simulink model "PMSM_FOC_Traction"  (R2020b)
settings: Solver=FixedStepAuto  StartTime=0.0  StopTime=10  RelTol=1e-3
model workspace (MAT data in the model file):
  wc : Simulink.Parameter (value not decoded)
values from neighbouring files (symbols this model uses):
  CL_Param = tmp_CL_Param    [PMSM_Parameters.m]
  Cosine_table = [1,0.999995293095708,0.999990587122738,0.999985881149769,0.999981174245477,0.999967055395246,0.999952936545014,0.999938818626106,0.999924698844552,0.999901168979704,0.999877639114857,0.999854108318687,0.999830577522516,0.999797635711730,0.999764694832265,0.999731753021479,0.999698810279369,0.999656459316611,0.999614108353853,0.999571758322418,0.999529405497015,0.999477646313608,0.999425887130201,0 ...(+75635 chars)    [Motor_Table.m]
  ctrlParamsPI = tmp_ctrlParamsPI    [PMSM_Parameters.m]
  Flux_weak = tmp_Fluxweak_struct    [PMSM_Parameters.m]
  FluxObsever = tmp_FluxObsever_struct    [PMSM_Parameters.m]
  Hall_Parameter = tmp_Hall_struct    [PMSM_Parameters.m]
  HFI = tmp_HFI_struct    [PMSM_Parameters.m]
  inverter = struct    [PMSM_Parameters.m]
  MTPA_id_table = [-1.39452500000000,-1.36697494250000,-1.33970177000000,-1.31270548250000,-1.28598608000000,-1.25954356250000,-1.23337793000000,-1.20748918250000,-1.18187732000000,-1.15654234250000,-1.13148425000000,-1.10670304250000,-1.08219872000000,-1.05797128250000,-1.03402073000000,-1.01034706250000,-0.986950280000000,-0.963830382500000,-0.940987370000000,-0.918421242500000,-0.896132000000000,-0.8741196425000 ...(+3439 chars)    [Motor_Table.m]
  MTPA_iq_table = [-10.2740250000000,-10.1791705677750,-10.0840783722000,-9.98875081492500,-9.89319029760000,-9.79739922187500,-9.70137998940000,-9.60513500182500,-9.50866666080000,-9.41197736797500,-9.31506952500000,-9.21794553352500,-9.12060779520000,-9.02305871167500,-8.92530068460000,-8.82733611562500,-8.72916740640000,-8.63079695857500,-8.53222717380000,-8.43346045372500,-8.33449920000000,-8.23534581427500,-8. ...(+3121 chars)    [Motor_Table.m]
  MTPA_Te_Max = single(1.50)    [Motor_Table.m]
  MTPA_Te_Min = single(-1.50)    [Motor_Table.m]
  OPL_Param = tmp_OPL_Param    [PMSM_Parameters.m]
  pmsm = struct    [PMSM_Parameters.m]
  Resolver_Parameter = tmp_Resolver_struct    [PMSM_Parameters.m]
  Sine_table = [0,0.00153398793190718,0.00306797679513693,0.00460196565836668,0.00613595545291901,0.00766988657414913,0.00920381769537926,0.0107377488166094,0.0122716808691621,0.0138054965063930,0.0153393121436238,0.0168731296434999,0.0184069443494082,0.0199405867606401,0.0214742291718721,0.0230078706517816,0.0245415139943361,0.0260749254375696,0.0276083368808031,0.0291417483240366,0.0306751597672701,0.032208281 ...(+75648 chars)    [Motor_Table.m]
  SMO = temp_SMO    [PMSM_Parameters.m]
undefined symbols (not defined in the file or in its folder): DiscIntNeverNeededParam, Kiv, Kiw, Kpv, Kpw, magnitude, sigbuilder_block, SVPWM, Vdc
libraries: powerlib x29, fl_lib x18, simulink x7, nesl_utility x7, pid_lib x5, dspstat3 x4, eeGeneralControl x4, eeDiscretePi x2, powerlib_extras x1, ee_lib x1
(part 3 of 6)

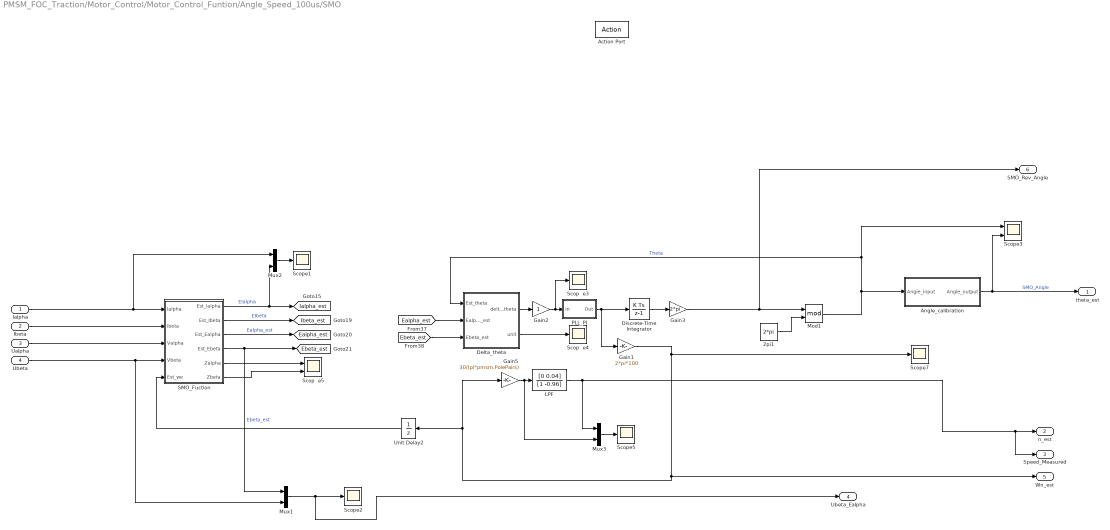
== system PMSM_FOC_Traction/Motor_Control/Motor_Control_Funtion/Angle_Speed_100us/SMO ==
  Ialpha : Inport
  Ibeta : Inport  Port=2
  Ualpha : Inport  Port=3
  Ubeta : Inport  Port=4
  Action Port : ActionPort  ActionPortLabel=if(u1==1)
  2pi1 : Constant  Value=2*pi  OutDataTypeStr=single
  Angle_calibration : Subsystem  TreatAsAtomicUnit=on
      settings: RTWSystemCode=Nonreusable function  RTWFcnNameOpts=Use subsystem name
  Delta_theta : Subsystem  TreatAsAtomicUnit=on
      settings: RTWSystemCode=Nonreusable function  RTWFcnNameOpts=Use subsystem name
  Discrete-Time Integrator : DiscreteIntegrator  gainval=100  SampleTime=-1  ICPrevOutput=DiscIntNeverNeededParam  ICPrevScaledInput=DiscIntNeverNeededParam
  Gain1 : Gain  Gain=2*pi*100  OutDataTypeStr=single
  Gain2 : Gain
  Gain3 : Gain  Gain=2*pi  OutDataTypeStr=single
  Gain5 : Gain  Gain=30/(pi*pmsm.PolePairs)
  LPF : DiscreteFilter  Numerator=[0 0.04]  Denominator=[1 -0.96]
  Mod1 : Math  Operator=mod  SaturateOnIntegerOverflow=on
  Mux1 : Mux  Inputs=2
  Mux2 : Mux  Inputs=2
  Mux3 : Mux  Inputs=2
  PLL_PI : Subsystem  mask{kp=SMO.PLL_KP, ki=SMO.PLL_Ki, Ts=-1}
  SMO_Fuction : Subsystem  mask{A=SMO.A, B=SMO.B, C=SMO.C, k=SMO.k, m=SMO.m, tao=SMO.tao, Ts=inverter.Ts}
  Scop  e3 : Scope
  Scop  e4 : Scope
  Scop  e5 : Scope  NumInputPorts=2
  Scope{1..2,5,7} (4 alike) : Scope
  Scope3 : Scope  NumInputPorts=2
  Unit Delay2 : UnitDelay  SampleTime=-1  HasFrameUpgradeWarning=on
  theta_est : Outport
  n_est : Outport  Port=2
  Speed_Measured : Outport  Port=3
  Ubeta_Ealpha : Outport  Port=4
  Wn_est : Outport  Port=5
  SMO_Rev_Angle : Outport  Port=6
  tag scope: Ealpha_est=global, Ebeta_est=global, Ialpha_est=global, Ibeta_est=global
  wires:
  SMO_Fuction/3(Est_Ealpha) -> [Ealpha_est]  "Ealpha_est"
  SMO_Fuction/6(Zbeta) -> Scop  e5/2
  SMO_Fuction/1(Est_Ialpha) -> Mux2/2, [Ialpha_est]  "EIalpha"
  SMO_Fuction/4(Est_Ebeta) -> Mux1/1, [Ebeta_est]  "Ebeta_est"
  SMO_Fuction/5(Zalpha) -> Scop  e5/1
  SMO_Fuction/2(Est_Ibeta) -> [Ibeta_est]  "EIbeta"
  Mux2/1 -> Scope1/1
  [Ebeta_est] -> Delta_theta/3(Ebeta_est)
  Delta_theta/1(delta_theta) -> Gain2/1
  Gain2/1 -> Scop  e3/1, PLL_PI/1(in)
  [Ealpha_est] -> Delta_theta/2(Ealpha_est)
  Discrete-Time Integrator/1 -> Gain3/1
  Mod1/1 -> Delta_theta/1(Est_theta), Scope3/1, Angle_calibration/1(Angle_input)  "Theta"
  PLL_PI/1(Out) -> Discrete-Time Integrator/1, Gain1/1
  2pi1/1 -> Mod1/2
  Mux3/1 -> Scope5/1
  Delta_theta/2(unit) -> Scop  e4/1
  Gain5/1 -> Mux3/2, LPF/1
  LPF/1 -> Speed_Measured/1, n_est/1, Mux3/1
  Angle_calibration/1(Angle_output) -> theta_est/1, Scope3/2  "SMO_Angle"
  Ialpha/1 -> SMO_Fuction/1(Ialpha), Mux2/1
  Ibeta/1 -> SMO_Fuction/2(Ibeta)
  Ualpha/1 -> SMO_Fuction/3(Valpha)
  Ubeta/1 -> SMO_Fuction/4(Vbeta), Mux1/2
  Gain1/1 -> Wn_est/1, Gain5/1, Unit Delay2/1, Scope7/1
  Mux1/1 -> Ubeta_Ealpha/1, Scope2/1
  Unit Delay2/1 -> SMO_Fuction/5(Est_we)
  Gain3/1 -> SMO_Rev_Angle/1, Mod1/1

== system PMSM_FOC_Traction/Motor_Control/Motor_Control_Funtion/Angle_Speed_100us/SpeedAndAngle ==
  Counter : Inport
  Hall : Inport  Port=2
  Action Port : ActionPort  ActionPortLabel=if(u1==1)
  ACC_OMG : Subsystem  TreatAsAtomicUnit=on
      settings: RTWSystemCode=Nonreusable function  RTWFcnNameOpts=Use subsystem name
  ADC_IRQ : Subsystem  TreatAsAtomicUnit=on
      settings: RTWSystemCode=Nonreusable function  RTWFcnNameOpts=Use subsystem name
  Chart : Stateflow chart  TreatAsAtomicUnit=on
  Scope : Scope
  Subsystem : Subsystem
  Subsystem1 : Subsystem
  Hall_Angle : Outport
  Hall_Speed_RPM : Outport  Port=2
  We : Outport  Port=3
  Gate : Outport  Port=4  VectorParamsAs1DForOutWhenUnconnected=off
  Duty : Outport  Port=5  VectorParamsAs1DForOutWhenUnconnected=off
  BLDC_State : Outport  Port=6  VectorParamsAs1DForOutWhenUnconnected=off
  wires:
  ACC_OMG/4(Counter) -> ADC_IRQ/4(Counter_Hall_IRQ)
  ACC_OMG/2(Acc) -> ADC_IRQ/2(Acc)
  ACC_OMG/3(OMG) -> [Hall_We], We/1, ADC_IRQ/3(OMG)
  ACC_OMG/1(Hall_SpeedRPM) -> Hall_Speed_RPM/1
  ACC_OMG/5(Six_theta) -> ADC_IRQ/5(Six_theta)
  Counter/1 -> ADC_IRQ/1(Counter_ADC_IRQ), ACC_OMG/1(Timer_Counter)
  ADC_IRQ/1(Hall_Angle) -> Hall_Angle/1, Scope/1
  Hall/1 -> Subsystem/2(Hall), ACC_OMG/2(Hall), ACC_OMG/Trigger
  Chart/1(BLDC_State) -> ACC_OMG/3(BLDC_State), Subsystem/1(BLDC_State), BLDC_State/1, Subsystem1/5(BLDC_State)
  Subsystem/2(Duty_Set) -> Subsystem1/2(Lock_Duty)
  ACC_OMG/6(Gate) -> Subsystem1/3(Hall_Gate)
  ACC_OMG/7(Tabc) -> Subsystem1/4(Hall_Duty)
  Subsystem/1(Gate) -> Subsystem1/1(Lock_Gate)
  Subsystem1/1(Gate) -> Gate/1
  Subsystem1/2(Tabc) -> Duty/1

== system PMSM_FOC_Traction/Motor_Control/Motor_Control_Funtion/Angle_Speed_100us/Speed_Angle_Selector ==
  Resolver_Speed : Inport
  Resolver_Angle : Inport  Port=2
  Resolver_PLL_Speed : Inport  Port=3
  Resolver_PLL_Angle : Inport  Port=4
  Sensorless_Speed : Inport  Port=5
  Sensorless_Angle : Inport  Port=6
  Hall_Speed : Inport  Port=7
  Hall_Angle : Inport  Port=8
  Hall : Subsystem
  Hall_Angle_Enable : Constant  Value=Hall_Parameter.Angle_Enable  OutDataTypeStr=uint8
  If1 : If  IfExpression=u1==1  ShowElse=off
  If2 : If  NumInputs=2  IfExpression=u1==1 | u2==1  ShowElse=off
  If3 : If  IfExpression=u1==1  ShowElse=off
  If5 : If  IfExpression=u1==1  ShowElse=off
  Merge : Merge  Inputs=4
  Merge1 : Merge  Inputs=4
  Resolver_Dir : Subsystem
  Resolver_Enable : Constant  Value=Resolver_Parameter.Angle_Enable  OutDataTypeStr=uint8
  Resolver_PLL : Subsystem
  Resolver_PLL_Enable : Constant  Value=Resolver_Parameter.PLL_Angle_Enable  OutDataTypeStr=uint8
  Sensorless : Subsystem
  Sensorless_Enable : Constant  Value=OPL_Param.Func_Enable  OutDataTypeStr=uint8
  Sensorless_Enable1 : Constant  Value=FluxObsever.Angle_Enable  OutDataTypeStr=uint8
  Speed : Outport
  Theta : Outport  Port=2
  wires:
  If5/1 -> Resolver_Dir/Action
  Resolver_Enable/1 -> If5/1
  Hall_Speed/1 -> Hall/1(In1)
  Hall_Angle/1 -> Hall/2(In2)
  Sensorless_Speed/1 -> Sensorless/1(In1)
  Sensorless_Angle/1 -> Sensorless/2(In2)
  Resolver_Speed/1 -> Resolver_Dir/1(In1)
  Resolver_Angle/1 -> Resolver_Dir/2(In2)
  Resolver_PLL_Speed/1 -> Resolver_PLL/1(In1)
  Resolver_PLL_Angle/1 -> Resolver_PLL/2(In2)
  If1/1 -> Resolver_PLL/Action
  Resolver_PLL_Enable/1 -> If1/1
  Sensorless_Enable/1 -> If2/1
  If2/1 -> Sensorless/Action
  Hall_Angle_Enable/1 -> If3/1
  If3/1 -> Hall/Action
  Resolver_Dir/1(Out1) -> Merge/1
  Resolver_PLL/1(Out1) -> Merge/2
  Sensorless/1(Out1) -> Merge/3
  Hall/1(Out1) -> Merge/4
  Resolver_Dir/2(Out2) -> Merge1/1
  Resolver_PLL/2(Out2) -> Merge1/2
  Sensorless/2(Out2) -> Merge1/3
  Hall/2(Out2) -> Merge1/4
  Merge1/1 -> Theta/1
  Merge/1 -> Speed/1
  Sensorless_Enable1/1 -> If2/2

== system PMSM_FOC_Traction/Motor_Control/Motor_Control_Funtion/Angle_Speed_100us/Speed_Resolver ==
  Theta : Inport
  Action Port : ActionPort  ActionPortLabel=if(u1==1)
  DT2 : DataTypeConversion  OutDataTypeStr=single
  Scope : Scope
  Scope1 : Scope
  Speed_cacl : Subsystem  TreatAsAtomicUnit=on
      settings: RTWSystemCode=Nonreusable function  RTWFcnNameOpts=Use subsystem name
  Speed_out : Outport
  Dir_Angle : Outport  Port=2
  wires:
  Theta/1 -> DT2/1, Speed_cacl/1(position)  "Theta_input"
  Speed_cacl/1(Speed_RPM) -> Scope1/1, Speed_out/1  "Speed_RPM_Filtered"
  DT2/1 -> Scope/1, Dir_Angle/1  "Direct_Angle"

== system PMSM_FOC_Traction/Motor_Control/Motor_Control_Funtion/Angle_Speed_100us/Startup_OPL ==
  OPL_Torque : Inport
  OPL_State : Inport  Port=2
  Smo_theta : Inport  Port=3
  Action Port : ActionPort  ActionPortLabel=if(u1==2|u1==3 | u1==3)
  If2 : If  IfExpression=u1==2  ElseIfExpressions=u1==3  ShowElse=off
  Merge : Merge
  Merge1 : Merge
  OPL_SpeedRPM : Constant  Value=OPL_Param.Target_RPM
  Scope3 : Scope  NumInputPorts=3
  Subsystem : Subsystem
  Subsystem1 : Subsystem
  Force_Angle : Outport
  OPL_Torque_Com : Outport  Port=2
  wires:
  OPL_State/1 -> If2/1
  If2/1 -> Subsystem/Action
  OPL_Torque/1 -> Subsystem1/1(OPL_Torque), Subsystem/2(OPL_Torque)
  If2/2 -> Subsystem1/Action
  Subsystem/1(Force_Angle) -> Merge/1
  Subsystem1/1(Force_Angle) -> Merge/2
  Merge/1 -> Force_Angle/1
  Subsystem/2(OPL_Torque_Com) -> Merge1/1
  Subsystem1/2(OPL_Torque_Com) -> Merge1/2
  Merge1/1 -> OPL_Torque_Com/1
  OPL_SpeedRPM/1 -> Subsystem1/3(Force_RPM), Subsystem/1(OPL_Speed)
  Smo_theta/1 -> Scope3/2, Subsystem/3(Smo_theta)
  Subsystem/3(Delta_theta) -> Subsystem1/2(Delta_theta)
  Subsystem/4(Force_Switch) -> Scope3/3, Subsystem1/4(Force_Switch)
  Subsystem1/3(Force_Angle1) -> Scope3/1

== system PMSM_FOC_Traction/Motor_Control/Motor_Control_Funtion/Angle_Speed_100us/Subsystem ==
  Action Port : ActionPort  ActionPortLabel=if((u1==1)&(u2==1))
  Sensorless_Enable : Constant  OutDataTypeStr=boolean
  Out1 : Outport
  wires:
  Sensorless_Enable/1 -> Out1/1

== system PMSM_FOC_Traction/Motor_Control/Motor_Control_Funtion/Angle_Speed_100us/Subsystem1 ==
  Action Port : ActionPort  ActionPortLabel=else
  Sensorless_Disable : Constant  Value=0  OutDataTypeStr=boolean
  Out1 : Outport
  wires:
  Sensorless_Disable/1 -> Out1/1

== system PMSM_FOC_Traction/Motor_Control/Motor_Control_Funtion/Control_Command_2ms/Speed_PI ==
  Speed_Command : Inport
  Speed_Measured : Inport  Port=2
  HFI_State : Inport  Port=3
  Motor_State : Inport  Port=4
  BLDC_State : Inport  Port=5
  Action Port : ActionPort  ActionPortLabel=case [ 1 ]:
  Add2 : Sum  Inputs=|+-
  Hall_Enalble : Constant  Value=Hall_Parameter.BLDC_Start  OutDataTypeStr=uint8
  If1 : If  NumInputs=2  IfExpression=(u1==1)&(u2==3)|(u1~=1)  ShowElse=off
  Scope2 : Scope
  Speed_PI : Subsystem
  Iq_ref : Outport  VectorParamsAs1DForOutWhenUnconnected=off
  wires:
  Speed_Command/1 -> Add2/1
  Speed_Measured/1 -> Add2/2
  Add2/1 -> Speed_PI/1(PI_input)  "currentControlError"
  Speed_PI/1(PI_out) -> Iq_ref/1, Scope2/1
  HFI_State/1 -> Speed_PI/2(HFI_State)
  Motor_State/1 -> Speed_PI/3(Motor_State)
  BLDC_State/1 -> If1/2
  Hall_Enalble/1 -> If1/1
  If1/1 -> Speed_PI/Action

== system PMSM_FOC_Traction/Motor_Control/Motor_Control_Funtion/Control_Command_2ms/Switch Case Action Subsystem ==
  Iq_in : Inport
  Action Port : ActionPort  ActionPortLabel=case [ 2 ]:
  Iq_out : Outport
  wires:
  Iq_in/1 -> Iq_out/1

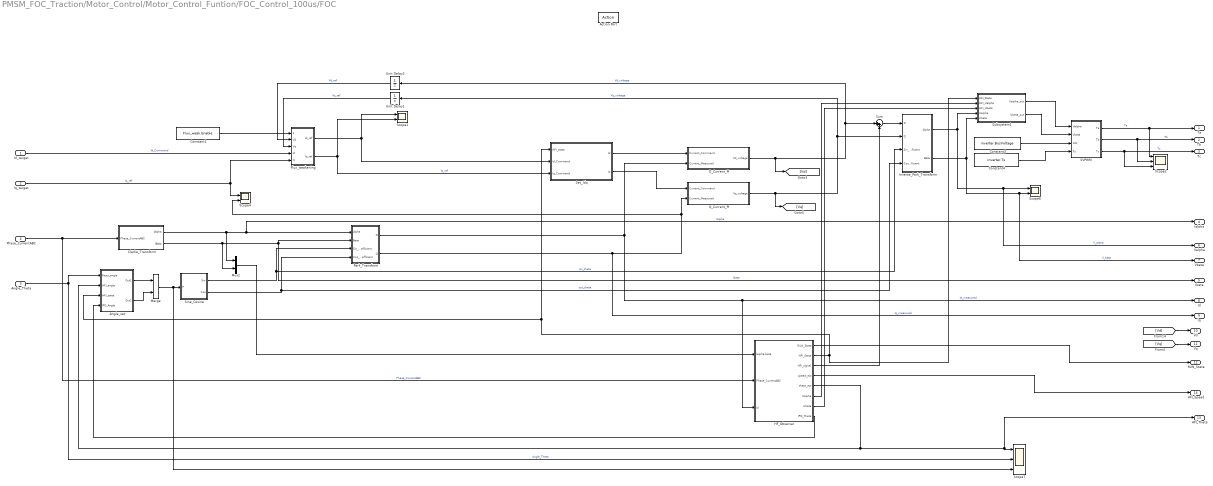
== system PMSM_FOC_Traction/Motor_Control/Motor_Control_Funtion/FOC_Control_100us/FOC ==
  Id_target : Inport
  Iq_target : Inport  Port=2
  Angle_Theta : Inport  Port=3  OutMin=0  OutMax=2*pi
  Phase_CurrentABC : Inport  Port=4  PortDimensions=3
  Action Port : ActionPort  ActionPortLabel=if((u1==1)&(u2==3)|(u1~=1))
  Angle_set : Subsystem  TreatAsAtomicUnit=on
      settings: RTWSystemCode=Nonreusable function  RTWFcnNameOpts=Use subsystem name
  Clarke_Transform : Subsystem  TreatAsAtomicUnit=on
      settings: RTWSystemCode=Nonreusable function  RTWFcnNameOpts=Use subsystem name
  Constant1 : Constant  Value=Flux_weak.Enable  OutDataTypeStr=single
  Constant3 : Constant  Value=inverter.BusVoltage  OutDataTypeStr=single
  Constant4 : Constant  Value=inverter.Ts  OutDataTypeStr=single
  D_Current_PI : Subsystem  TreatAsAtomicUnit=on
      settings: RTWSystemCode=Nonreusable function  RTWFcnNameOpts=Use subsystem name
  "Flux_weakening " : Subsystem
  HF_Observer : Subsystem  TreatAsAtomicUnit=on
      settings: RTWSystemCode=Nonreusable function  RTWFcnNameOpts=Use subsystem name  RTWFileNameOpts=Use subsystem name
  Inverse_Park_Transform : Subsystem  TreatAsAtomicUnit=on
      settings: RTWSystemCode=Nonreusable function  RTWFcnNameOpts=Use subsystem name
      mask Display:
      | port_label('input',1,'D')
      | port_label('input',2,'Q')
      | port_label('input',3,'Sin')
      | port_label('input',4,'Cos')
      | port_label('output',1,'\alpha','texmode', 'on')
      | port_label('output',2,'\beta','texmode', 'on')
  Merge : Merge
  Mux2 : Mux  Inputs=2
  Park_Transform : Subsystem  TreatAsAtomicUnit=on
      settings: RTWSystemCode=Nonreusable function  RTWFcnNameOpts=Use subsystem name
      mask Display:
      | port_label('input',1,'\alpha','texmode', 'on')
      | port_label('input',2,'\beta','texmode', 'on')
      | port_label('input',3,'Sin')
      | port_label('input',4,'Cos')
      | port_label('output',1,'D')
      | port_label('output',2,'Q')
  Q_Current_PI : Subsystem  TreatAsAtomicUnit=on
      settings: RTWSystemCode=Nonreusable function  RTWFcnNameOpts=Use subsystem name
  SVPWM : Subsystem  AncestorBlock=SVPWM/SVPWM  TreatAsAtomicUnit=on  RTWFcnName=SVPWM  RTWFileName=SVPWM
      settings: RTWSystemCode=Nonreusable function  RTWFcnNameOpts=Use subsystem name
      mask Display:
      | plot([0.000 0.020 0.041 0.061 0.082 0.102 0.122 0.143 0.163 0.184 0.204 0.224 0.245 0.265 0.286 0.306 0.327 0.347 0.367 0.388 0.408 0.429 0.449 0.469 0.490 0.510 0.531 0.551 0.571 0.592 0.612 0.633 0.653 0.673 0.694 0.714 0.735 0.755 0.776 0.796 0.816 0.837 0.857 0.878 0.898 0.918 0.939 0.959 0.980 1.000 ], ...
      |      [0.500 0.586 0.671 0.753 0.831 0.858 0.875 0.885 0.890 0.887 0.879 0.864 0.844 0.855 0.872 0.884 0.889 0.888 0.881 0.867 0.847 0.793 0.713 0.629 0.543 0.457 0.371 0.287 0.207 0.153 0.133 0.119 0.112 0.111 0.116 0.128 0.145 0.156 0.136 0.121 0.113 0.110 0.115 0.125 0.142 0.169 0.247 0.329 0.414 0.500 ])
  Scope1 : Scope  NumInputPorts=2
  Scope2 : Scope  NumInputPorts=3
  Scope4 : Scope  NumInputPorts=2
  Scope6 : Scope  NumInputPorts=2
  Scope7 : Scope  NumInputPorts=3
  Set_Idq : Subsystem  TreatAsAtomicUnit=on
      settings: RTWSystemCode=Nonreusable function  RTWFcnNameOpts=Use subsystem name
  Sine_Cosine : Subsystem  TreatAsAtomicUnit=on
      settings: RTWSystemCode=Nonreusable function  RTWFcnNameOpts=Use subsystem name
  Subsystem1 : Subsystem
  Sum : Sum  Inputs=|++
  Unit Delay1 : UnitDelay  SampleTime=-1  HasFrameUpgradeWarning=on
  Unit Delay2 : UnitDelay  SampleTime=-1  HasFrameUpgradeWarning=on
  Ta : Outport
  Tb : Outport  Port=2
  Tc : Outport  Port=3
  Ialpha : Outport  Port=4
  Ibeta : Outport  Port=5
  Valpha : Outport  Port=6
  Vbeta : Outport  Port=7
  Id : Outport  Port=8
  Iq : Outport  Port=9
  Vd : Outport  Port=10
  Vq : Outport  Port=11
  RUN_State : Outport  Port=12
  HFI_Theta : Outport  Port=13
  HFI_Speed : Outport  Port=14
  wires:
  Park_Transform/1(D) -> HF_Observer/3(Id), Id/1, D_Current_PI/2(Current_Measured)  "Id_measured"
  Constant4/1 -> SVPWM/4(Ts)
  SVPWM/3(Tc) -> Tc/1, Scope2/3  "Tc"
  SVPWM/2(Tb) -> Scope2/2, Tb/1  "Tb"
  Park_Transform/2(Q) -> Iq/1, Scope4/2, Q_Current_PI/2(Current_Measured)  "Iq_measured"
  Sine_Cosine/2(Cos) -> Park_Transform/4(Cos_Coefficient), Inverse_Park_Transform/4(Cos_Coefficient)  "cos_theta"
  Sine_Cosine/1(Sin) -> Park_Transform/3(Sin_Coefficient), Inverse_Park_Transform/3(Sin_Coefficient)  "sin_theta"
  Constant3/1 -> SVPWM/3(Vdc)
  D_Current_PI/1(Vd_voltage) -> [Vd], Unit Delay2/1, Sum/1  "Vd_voltage"
  Q_Current_PI/1(Vq_voltage) -> [Vq], Unit Delay1/1, Inverse_Park_Transform/2(Q)  "Vq_voltage"
  SVPWM/1(Ta) -> Scope2/1, Ta/1  "Ta"
  Id_target/1 -> "Flux_weakening "/4(Id)  "Id_Command"
  Iq_target/1 -> "Flux_weakening "/5(Iq), Scope4/1  "Iq_ref"
  Clarke_Transform/2(IBeta) -> Mux2/2, Ibeta/1, Park_Transform/2(Beta)  "Ibeta"
  Clarke_Transform/1(IAlpha) -> Ialpha/1, Park_Transform/1(Alpha), Mux2/1  "Ialpha"
  Unit Delay2/1 -> "Flux_weakening "/2(Vd)  "Vd_ref"
  Unit Delay1/1 -> "Flux_weakening "/3(Vq)  "Vq_ref"
  "Flux_weakening "/1(Id_ref) -> Scope1/1, Set_Idq/2(Id_Command)
  "Flux_weakening "/2(Iq_ref) -> Set_Idq/3(Iq_Command), Scope1/2  "Iq_ref"
  Constant1/1 -> "Flux_weakening "/1(Enable)
  Inverse_Park_Transform/1(Alpha) -> Scope6/1, Valpha/1, Subsystem1/4(Ualpha)  "V_alpha"
  Inverse_Park_Transform/2(Beta) -> Scope6/2, Vbeta/1, Subsystem1/5(Ubeta)  "V_beta"
  Phase_CurrentABC/1 -> HF_Observer/2(Phase_CurrentABC), Clarke_Transform/1(Phase_CurrentABC)  "Phase_CurrentABC"
  Sum/1 -> Inverse_Park_Transform/1(D)
  HF_Observer/3(HFI_signal) -> Sum/2
  HF_Observer/4(speed_est) -> HFI_Speed/1
  Angle_Theta/1 -> Scope7/2, Angle_set/1(Reso_angle)  "Angle_Theta"
  Mux2/1 -> HF_Observer/1(Ialpha-beta)
  HF_Observer/5(theta_est) -> HFI_Theta/1, Scope7/1, Angle_set/2(HFI_angle)
  Merge/1 -> Scope7/3, Sine_Cosine/1(P)
  Angle_set/1(Out1) -> Merge/1
  Angle_set/2(Out2) -> Merge/2
  Subsystem1/1(Ualpha_out) -> SVPWM/1(Valpha)
  Subsystem1/2(Ubeta_out) -> SVPWM/2(Vbeta)
  HF_Observer/6(Ualpha) -> Subsystem1/2(HFI_Ualpha)
  HF_Observer/7(Ubeta) -> Subsystem1/3(HFI_Ubeta)
  HF_Observer/2(HFI_State) -> Subsystem1/1(HFI_State), Set_Idq/1(HFI_state), Angle_set/3(HFI_state)
  HF_Observer/1(RUN_State) -> RUN_State/1
  Set_Idq/1(Id) -> D_Current_PI/1(Current_Command)
  Set_Idq/2(Iq) -> Q_Current_PI/1(Current_Command)
  HF_Observer/8(IPD_Theta) -> Angle_set/4(IPD_Angle)
  [Vq] -> Vq/1
  [Vd] -> Vd/1

== system PMSM_FOC_Traction/Motor_Control/Motor_Control_Funtion/FOC_Control_100us/Iq_selector ==
  Motor_state : Inport
  PI_IQ : Inport  Port=2
  OPL_IQ : Inport  Port=3
  If1 : If  IfExpression=u1 ==2 | u1 ==3
  Merge : Merge
  Subsystem : Subsystem
  Subsystem1 : Subsystem
  Iq_ref : Outport
  wires:
  Motor_state/1 -> If1/1
  If1/1 -> Subsystem/Action
  OPL_IQ/1 -> Subsystem/1(In1)
  PI_IQ/1 -> Subsystem1/1(In1)
  Subsystem/1(Out1) -> Merge/1
  Subsystem1/1(Out1) -> Merge/2
  Merge/1 -> Iq_ref/1
  If1/2 -> Subsystem1/Action

== system PMSM_FOC_Traction/Motor_Control/Motor_Control_Funtion/FOC_Control_100us/MTPA ==
  Te_ref : Inport
  1-D Lookup Table4 : Lookup_n-D  NumberOfTableDimensions=1  LookupTableObject=''  BreakpointsForDimension1=single(linspace(MTPA_Te_Min,MTPA_Te_Max,length(MTPA_id_table)));  BreakpointsForDimension1FirstPoint=10  BreakpointsForDimension2FirstPoint=10  BreakpointsForDimension1Spacing=12  BreakpointsForDimension2Spacing=12  IndexSearchMethod=Evenly spaced points  Table=MTPA_id_table  InterpMethod=Flat  DiagnosticForOutOfRangeInput=Error  InternalRulePriority=Speed  RndMeth=Simplest  InputSameDT=on
  1-D Lookup Table5 : Lookup_n-D  NumberOfTableDimensions=1  LookupTableObject=''  BreakpointsForDimension1=single(linspace(MTPA_Te_Min,MTPA_Te_Max,length(MTPA_id_table)));  BreakpointsForDimension1FirstPoint=10  BreakpointsForDimension2FirstPoint=10  BreakpointsForDimension1Spacing=12  BreakpointsForDimension2Spacing=12  IndexSearchMethod=Evenly spaced points  Table=MTPA_iq_table  InterpMethod=Flat  DiagnosticForOutOfRangeInput=Error  InternalRulePriority=Speed  RndMeth=Simplest  InputSameDT=on
  Saturation : Saturate  UpperLimit=MTPA_Te_Max-0.01  LowerLimit=MTPA_Te_Min+0.01
  Saturation1 : Saturate  UpperLimit=MTPA_Te_Max-0.01  LowerLimit=MTPA_Te_Min+0.01
  Id_ref : Outport
  Iq_ref : Outport  Port=2
  wires:
  Te_ref/1 -> Saturation1/1, Saturation/1
  Saturation/1 -> 1-D Lookup Table4/1
  Saturation1/1 -> 1-D Lookup Table5/1
  1-D Lookup Table4/1 -> Id_ref/1
  1-D Lookup Table5/1 -> Iq_ref/1

== system PMSM_FOC_Traction/Motor_Control/Motor_Control_Funtion/Motor_State_10ms/Power_Cacl ==
  Id : Inport
  Vd : Inport  Port=2
  Iq : Inport  Port=3
  Vq : Inport  Port=4
  Add : Sum
  Product : Product
  Product1 : Product
  Power : Outport
  wires:
  Id/1 -> Product/1
  Vd/1 -> Product/2
  Iq/1 -> Product1/1
  Vq/1 -> Product1/2
  Product/1 -> Add/1
  Product1/1 -> Add/2
  Add/1 -> Power/1

== system PMSM_FOC_Traction/Motor_Control/Motor_Control_Funtion/Motor_State_10ms/Torque_Cacl ==
  Id : Inport
  Iq : Inport  Port=2
  Constant : Constant  Value=3/2  OutDataTypeStr=single
  Constant1 : Constant  Value=pmsm.PolePairs  OutDataTypeStr=single
  Constant2 : Constant  Value=pmsm.FluxLinkage  OutDataTypeStr=single
  Constant3 : Constant  Value=pmsm.InductanceLd  OutDataTypeStr=single
  Constant4 : Constant  Value=pmsm.InductanceLq  OutDataTypeStr=single
  Product{,1..4} (5 alike) : Product
  Subtract : Sum
  Subtract1 : Sum  Inputs=+-
  Torque : Outport
  wires:
  Constant1/1 -> Product/1
  Constant/1 -> Product/2
  Constant2/1 -> Product1/1
  Iq/1 -> Product1/2, Product3/1
  Product1/1 -> Subtract/1
  Constant3/1 -> Subtract1/1
  Constant4/1 -> Subtract1/2
  Subtract1/1 -> Product2/1
  Id/1 -> Product2/2
  Product2/1 -> Product3/2
  Product3/1 -> Subtract/2
  Product/1 -> Product4/1
  Subtract/1 -> Product4/2
  Product4/1 -> Torque/1

== system PMSM_FOC_Traction/PMSM/Control/Control/Commutation ==
  Hall : Inport
  Bias : Bias  Bias=-1
  Bit concatenate : Subsystem
  Data Type Conversion : DataTypeConversion
  Direct Lookup Table (n-D)2 : LookupNDDirect  InputsSelectThisObjectFromTable=Vector  Table=[0 0 0 1 1 0;0 1 1 0 0 0;0 1 0 0 0 1;1 0 0 0 1 0;1 0 1 0 0 0;0 0 0 1 0 1]
  S : Outport  VectorParamsAs1DForOutWhenUnconnected=off
  wires:
  Hall/1 -> Bit concatenate/1(u)
  Bit concatenate/1(y) -> Data Type Conversion/1
  Direct Lookup Table (n-D)2/1 -> S/1
  Data Type Conversion/1 -> Bias/1
  Bias/1 -> Direct Lookup Table (n-D)2/1

== system PMSM_FOC_Traction/PMSM/SpeedAndAngle/ACC_OMG/Six_point ==
  In1 : Inport
  Merge2 : Merge  Inputs=6
  Scope : Scope  NumInputPorts=2
  Sector_1 : Subsystem
  Sector_2 : Subsystem
  Sector_3 : Subsystem
  Sector_4 : Subsystem
  Sector_5 : Subsystem
  Sector_6 : Subsystem
  Switch Case2 : SwitchCase  CaseConditions={1,2,3,4,5,6}  ShowDefaultCase=off
  Out1 : Outport
  wires:
  Sector_4/1(Angle_0) -> Merge2/4
  Switch Case2/5 -> Sector_5/Action
  Sector_6/1(Angle_0) -> Merge2/6
  Sector_5/1(Angle_0) -> Merge2/5
  Switch Case2/6 -> Sector_6/Action
  Switch Case2/3 -> Sector_3/Action
  Switch Case2/4 -> Sector_4/Action
  Sector_1/1(Angle_0) -> Merge2/1
  Switch Case2/2 -> Sector_2/Action
  In1/1 -> Scope/1, Switch Case2/1
  Sector_3/1(Angle_0) -> Merge2/3
  Switch Case2/1 -> Sector_1/Action
  Sector_2/1(Angle_0) -> Merge2/2
  Merge2/1 -> Scope/2, Out1/1

== system PMSM_FOC_Traction/PMSM/SpeedAndAngle/ADC_IRQ/HallAngle_calibration ==
  Angle_input : Inport
  Angle_offset : Constant  Value=SMO.Angle_offset
  If Action Subsystem1 : Subsystem  TreatAsAtomicUnit=on
  If Action Subsystem2 : Subsystem  TreatAsAtomicUnit=on
  If Action Subsystem3 : Subsystem  TreatAsAtomicUnit=on
  If1 : If  IfExpression=u1 > 6.283185307  ElseIfExpressions=u1<0
  Merge1 : Merge  Inputs=3
  Subtract1 : Sum
  Angle_output : Outport
  wires:
  Angle_input/1 -> Subtract1/1
  Angle_offset/1 -> Subtract1/2  "Control_ModeCommand"
  If1/1 -> If Action Subsystem2/Action
  If1/3 -> If Action Subsystem1/Action
  If Action Subsystem2/1(Out1) -> Merge1/1
  Subtract1/1 -> If Action Subsystem3/1(In1), If Action Subsystem1/1(In1), If Action Subsystem2/1(In1), If1/1
  If Action Subsystem1/1(Out1) -> Merge1/3
  If Action Subsystem3/1(Out1) -> Merge1/2
  If1/2 -> If Action Subsystem3/Action
  Merge1/1 -> Angle_output/1

== system PMSM_FOC_Traction/Motor_Control/Motor_Control_Funtion/Angle_Speed_100us/Angle_Selector/Subsystem ==
  In1 : Inport
  Action Port : ActionPort  ActionPortLabel=if(u1 ==2 | u1 ==3)
  Out1 : Outport
  wires:
  In1/1 -> Out1/1

== system PMSM_FOC_Traction/Motor_Control/Motor_Control_Funtion/Angle_Speed_100us/Angle_Selector/Subsystem1 ==
  In1 : Inport
  Action Port : ActionPort  ActionPortLabel=elseif(u1 ==4)
  Out1 : Outport
  wires:
  In1/1 -> Out1/1

== system PMSM_FOC_Traction/Motor_Control/Motor_Control_Funtion/Angle_Speed_100us/Flux_OBSERVER/equ3.12 ==
  eta_x1_hat : Inport  OutDataTypeStr=single
  eta_x2_hat : Inport  Port=2  OutDataTypeStr=single
  Constant : Constant  Value=FluxObsever.Omega  OutDataTypeStr=single  SampleTime=-1
  Discrete PID Controller : pid_lib/PID Controller  Controller=PI  Form=Parallel  TimeDomain=Discrete-time  UseExternalTs=off  SampleTime=-1  IntegratorMethod=Forward Euler  FilterMethod=Forward Euler  ControllerParametersSource=external  P=2*0.707*1650  I=1650*1650  D=0  UseFilter=on  N=100  TunerSelectOption=Transfer Function Based (PID Tuner App)  ZeroCross=off  InitialConditionSource=internal  InitialConditionForIntegrator=0  InitialConditionForFilter=0  DifferentiatorICPrevScaledInput=0  ExternalReset=none  TrackingMode=off  Kt=1  LimitOutput=on  SatLimitsSource=internal  UpperSaturationLimit=2500*2*pi*pmsm.PolePairs/60  LowerSaturationLimit=-2500*2*pi*pmsm.PolePairs/60  LinearizeAsGain=off  AntiWindupMode=clamping  Kb=1  POutMin=[]  POutMax=[]  IOutMin=[]  IOutMax=[]  DOutMin=[]  DOutMax=[]  NOutMin=[]  NOutMax=[]  SumOutMin=[]  SumOutMax=[]  SaturationOutMin=[]  SaturationOutMax=[]  PParamMin=[]  PParamMax=[]  IParamMin=[]  IParamMax=[]  DParamMin=[]  DParamMax=[]  NParamMin=[]  NParamMax=[]  KbParamMin=[]  KbParamMax=[]  KtParamMin=[]  KtParamMax=[]  KbOutMin=[]  KbOutMax=[]  KtOutMin=[]  KtOutMax=[]  IntegratorOutMin=[]  IntegratorOutMax=[]  FilterOutMin=[]  FilterOutMax=[]  SumI1OutMin=[]  SumI1OutMax=[]  SumI2OutMin=[]  SumI2OutMax=[]  SumI3OutMin=[]  SumI3OutMax=[]  SumI4OutMin=[]  SumI4OutMax=[]  SumDOutMin=[]  SumDOutMax=[]  DifferentiatorOutMin=[]  DifferentiatorOutMax=[]  FilterDiffOutCoefMin=[]  FilterDiffOutCoefMax=[]  ReciprocalOutMin=[]  ReciprocalOutMax=[]  SumDenOutMin=[]  SumDenOutMax=[]  SumNumOutMin=[]  SumNumOutMax=[]  DivideOutMin=[]  DivideOutMax=[]  UdiffTsProdOutMin=[]  UdiffTsProdOutMax=[]  NTsProdOutMin=[]  NTsProdOutMax=[]  UintegralTsProdOutMin=[]  UintegralTsProdOutMax=[]  UngainTsProdOutMin=[]  UngainTsProdOutMax=[]  IntegratorContinuousStateAttributes=''  IntegratorStateMustResolveToSignalObject=off  IntegratorRTWStateStorageClass=Auto  FilterContinuousStateAttributes=''  FilterStateMustResolveToSignalObject=off  FilterRTWStateStorageClass=Auto  ParallelPVariant=ExternalParameters  IdealPVariant=Disabled  IVariant=ExternalParameters  DVariant=Disabled  IntegratorVariant=Discrete  SatVariant=Enabled  AWVariant=DiscClampingParallel  PCopyVariant=Disabled  TRVariant=Disabled  FdbkBlocksVariant=Forward  IdealPFdbkVariant=Disabled  SatFdbkVariant=Disabled  DerivativeFilterVariant=Disabled  NVariant=Disabled  NCopyVariant=Disabled_SignalSpec  FilterICVariant=Disabled  IntegratorICVariant=InternalICs  ExternalResetVariant=Disabled  TRSumVariant=Passthrough  SumFdbkVariant=Disabled  SumVariant=Sum_PI  TsampFilterVariant=InternalTs  TsampNgainVariant=Passthrough  TsampIntegralVariant=Passthrough  ExternalSaturationOutDataTypeStr=Inherit: Same as second input
  Gain : Gain  Gain=FluxObsever.Kp  OutDataTypeStr=single
  Product : Product  OutDataTypeStr=single
  Product1 : Product  OutDataTypeStr=single
  Product2 : Product  OutDataTypeStr=single
  Sine_Cosine : Subsystem  TreatAsAtomicUnit=on
      settings: RTWSystemCode=Nonreusable function  RTWFcnNameOpts=Use subsystem name
  Sum : Sum  Inputs=-|+  OutDataTypeStr=single
  integrator : Subsystem
  Theta : Outport  OutDataTypeStr=single
  omega_e_hat : Outport  Port=2  OutDataTypeStr=single
  wires:
  Product/1 -> Sum/1
  Product1/1 -> Sum/2
  Sum/1 -> Discrete PID Controller/1
  Sine_Cosine/2(Cos) -> Product1/2
  Sine_Cosine/1(Sin) -> Product/1
  integrator/1(y(k-1)) -> Sine_Cosine/1(P), Theta/1  "ObserverTheta"
  eta_x1_hat/1 -> Product/2
  eta_x2_hat/1 -> Product1/1
  Gain/1 -> Discrete PID Controller/2
  Constant/1 -> Product2/2, Product2/1, Gain/1
  Product2/1 -> Discrete PID Controller/3
  Discrete PID Controller/1 -> omega_e_hat/1, integrator/1(x(k))

== system PMSM_FOC_Traction/Motor_Control/Motor_Control_Funtion/Angle_Speed_100us/Flux_OBSERVER/equ3.6 ==
  i_alpha : Inport  OutDataTypeStr=single
  u_alpha : Inport  Port=2  OutDataTypeStr=single
  i_beta : Inport  Port=3  OutDataTypeStr=single
  u_beta : Inport  Port=4  OutDataTypeStr=single
  omega_e_hat : Inport  Port=5  OutDataTypeStr=single
  Add4 : Sum  Inputs=-+  OutDataTypeStr=single
  Add5 : Sum  Inputs=-+  OutDataTypeStr=single
  Gain : Gain  Gain=0.005  OutDataTypeStr=single
  Gain1 : Gain  Gain=pmsm.StatorPhaseResistance  OutDataTypeStr=single
  Product : Product  OutDataTypeStr=single
  Product1 : Product  OutDataTypeStr=single
  Saturation : Saturate  UpperLimit=1  LowerLimit=0.8  OutDataTypeStr=single
  y1 : Outport  OutDataTypeStr=single
  y2 : Outport  Port=2  OutDataTypeStr=single
  wires:
  Add5/1 -> y2/1
  Product/1 -> Add4/1
  Product1/1 -> Add5/1
  u_beta/1 -> Add5/2
  i_beta/1 -> Product1/1
  Add4/1 -> y1/1
  i_alpha/1 -> Product/1
  u_alpha/1 -> Add4/2
  Gain/1 -> Saturation/1
  Saturation/1 -> Gain1/1
  omega_e_hat/1 -> Gain/1
  Gain1/1 -> Product/2, Product1/2

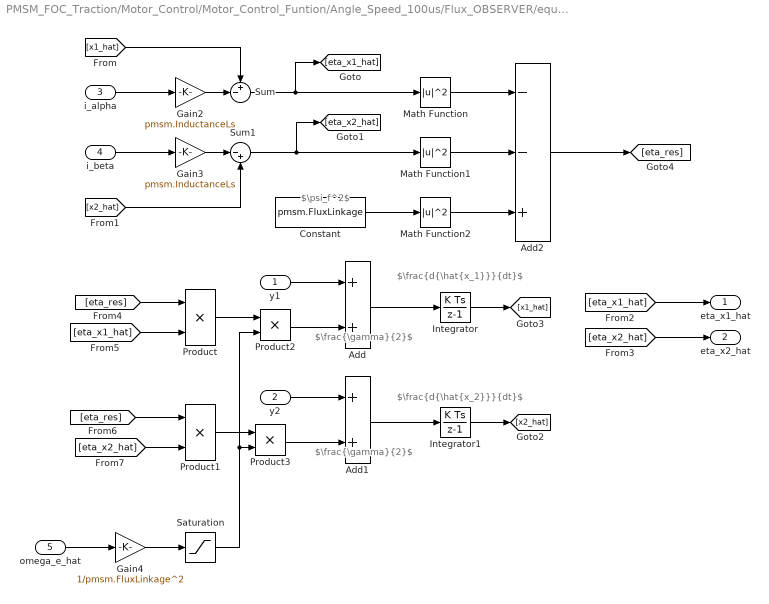
== system PMSM_FOC_Traction/Motor_Control/Motor_Control_Funtion/Angle_Speed_100us/Flux_OBSERVER/equ3.9 ==
  note: $\frac{d{\hat{x_1}}}{dt}$
  note: $\frac{d{\hat{x_2}}}{dt}$
  note: $\frac{\gamma}{2}$
  note: $\frac{\gamma}{2}$
  note: $\psi_f^2$
  y1 : Inport  OutDataTypeStr=single
  y2 : Inport  Port=2  OutDataTypeStr=single
  i_alpha : Inport  Port=3  OutDataTypeStr=single
  i_beta : Inport  Port=4  OutDataTypeStr=single
  omega_e_hat : Inport  Port=5  OutDataTypeStr=single
  Add : Sum  OutDataTypeStr=single
  Add1 : Sum  OutDataTypeStr=single
  Add2 : Sum  Inputs=--+  OutDataTypeStr=single
  Constant : Constant  Value=pmsm.FluxLinkage  OutDataTypeStr=single
  Gain2 : Gain  Gain=pmsm.InductanceLs  OutDataTypeStr=single
  Gain3 : Gain  Gain=pmsm.InductanceLs  OutDataTypeStr=single
  Gain4 : Gain  Gain=1/pmsm.FluxLinkage^2  OutDataTypeStr=single
  Integrator : DiscreteIntegrator  SampleTime=-1  OutDataTypeStr=single  ICPrevOutput=DiscIntNeverNeededParam  ICPrevScaledInput=DiscIntNeverNeededParam  mask(DiscretizedDiscreteIntegrator){}
      mask init:
      | %zoh
  Integrator1 : DiscreteIntegrator  SampleTime=-1  OutDataTypeStr=single  ICPrevOutput=DiscIntNeverNeededParam  ICPrevScaledInput=DiscIntNeverNeededParam  mask(DiscretizedDiscreteIntegrator){}
      mask init:
      | %zoh
  Math Function : Math  Operator=magnitude^2  OutDataTypeStr=single  SaturateOnIntegerOverflow=on
  Math Function1 : Math  Operator=magnitude^2  OutDataTypeStr=single  SaturateOnIntegerOverflow=on
  Math Function2 : Math  Operator=magnitude^2  OutDataTypeStr=single  SaturateOnIntegerOverflow=on
  Product{,1..3} (4 alike) : Product  OutDataTypeStr=single
  Saturation : Saturate  UpperLimit=500e4  LowerLimit=20e4  OutDataTypeStr=single
  Sum : Sum  Inputs=+-|  OutDataTypeStr=single
  Sum1 : Sum  Inputs=|-+  OutDataTypeStr=single
  eta_x1_hat : Outport  OutDataTypeStr=single
  eta_x2_hat : Outport  Port=2  OutDataTypeStr=single
  wires:
  y1/1 -> Add/1
  Product3/1 -> Add1/2
  Product1/1 -> Product3/1
  Sum/1 -> [eta_x1_hat], Math Function/1
  Product/1 -> Product2/1
  Product2/1 -> Add/2
  Add/1 -> Integrator/1
  Add1/1 -> Integrator1/1
  Sum1/1 -> Math Function1/1, [eta_x2_hat]
  Integrator1/1 -> [x2_hat]
  y2/1 -> Add1/1
  Integrator/1 -> [x1_hat]
  i_beta/1 -> Gain3/1
  i_alpha/1 -> Gain2/1
  [x2_hat] -> Sum1/2
  Gain3/1 -> Sum1/1
  Math Function1/1 -> Add2/2
  Gain2/1 -> Sum/2
  [x1_hat] -> Sum/1
  Math Function/1 -> Add2/1
  Add2/1 -> [eta_res]
  [eta_x1_hat] -> eta_x1_hat/1
  [eta_x2_hat] -> eta_x2_hat/1
  [eta_res] -> Product/1
  [eta_x1_hat] -> Product/2
  [eta_res] -> Product1/1
  [eta_x2_hat] -> Product1/2
  Constant/1 -> Math Function2/1
  Math Function2/1 -> Add2/3
  omega_e_hat/1 -> Gain4/1
  Gain4/1 -> Saturation/1
  Saturation/1 -> Product2/2, Product3/2

== system PMSM_FOC_Traction/Motor_Control/Motor_Control_Funtion/Angle_Speed_100us/HIGH_SMO/Equ1 ==
  note: i_alpha_hat(k)
  note: GainK/Ld
  note: i_alpha_hat
  note: R/Ld
  note: (Ld-Lq)/Ld
  note: i_alpha_hat_dot
  note: 1/Ld
  note: e_alpha_hat
  note: 1/Ld
  note: i_beta_hat
  note: Omega_hat
  note: i_alpha_hat(k-1)
  omega_hat : Inport
  e_alpha_hat : Inport  Port=2
  u_alpha : Inport  Port=3
  I_beta_hat : Inport  Port=4
  alpha_err : Inport  Port=5
  Add : Sum  Inputs=---+-
  Gain : Gain  Gain=pmsm.StatorPhaseResistance/pmsm.InductanceLd
  Gain1 : Gain  Gain=(pmsm.InductanceLd-pmsm.InductanceLq)/pmsm.InductanceLd
  Gain17 : Gain  Gain=1/pmsm.InductanceLd
  Gain2 : Gain  Gain=1/pmsm.InductanceLd
  Gain4 : Gain  Gain=SMO.k/pmsm.InductanceLd
  Integrator : DiscreteIntegrator  IntegratorMethod=Integration: Backward Euler  SampleTime=-1  ICPrevOutput=DiscIntNeverNeededParam  ICPrevScaledInput=DiscIntNeverNeededParam  mask(DiscretizedDiscreteIntegrator){}
      mask init:
      | %tustin
  Product : Product
  Unit Delay : UnitDelay  SampleTime=-1  HasFrameUpgradeWarning=on
  i_alpha_hat : Outport
  wires:
  Gain1/1 -> Add/2
  Gain4/1 -> Add/5
  Product/1 -> Gain1/1
  Add/1 -> Integrator/1
  I_beta_hat/1 -> Product/1
  Unit Delay/1 -> [i_alpha_hat], i_alpha_hat/1
  Gain/1 -> Add/1
  u_alpha/1 -> Gain2/1
  Gain2/1 -> Add/4
  Integrator/1 -> Unit Delay/1
  omega_hat/1 -> Product/2
  Gain17/1 -> Add/3
  e_alpha_hat/1 -> Gain17/1
  alpha_err/1 -> Gain4/1
  [i_alpha_hat] -> Gain/1

== system PMSM_FOC_Traction/Motor_Control/Motor_Control_Funtion/Angle_Speed_100us/HIGH_SMO/Equ2 ==
  note: R/Ld
  note: (Ld-Lq)/Ld
  note: 1/Ld
  note: i_alpha_hat
  note: Omega_hat
  note: 1/Ld
  note: GainK/Ld
  note: i_beta_hat_dot
  omega_hat : Inport
  i_alpha_hat : Inport  Port=2
  e_beta_hat : Inport  Port=3
  u_beta : Inport  Port=4
  beta_err : Inport  Port=5
  Add1 : Sum  Inputs=+--+-
  Gain3 : Gain  Gain=1/pmsm.InductanceLd
  Gain5 : Gain  Gain=1/pmsm.InductanceLd
  Gain6 : Gain  Gain=SMO.k/pmsm.InductanceLd
  Gain7 : Gain  Gain=(pmsm.InductanceLd-pmsm.InductanceLq)/pmsm.InductanceLd
  Gain8 : Gain  Gain=pmsm.StatorPhaseResistance/pmsm.InductanceLd
  Integrator1 : DiscreteIntegrator  IntegratorMethod=Integration: Backward Euler  SampleTime=-1  ICPrevOutput=DiscIntNeverNeededParam  ICPrevScaledInput=DiscIntNeverNeededParam  mask(DiscretizedDiscreteIntegrator){}
      mask init:
      | %tustin
  Product1 : Product
  Unit Delay1 : UnitDelay  SampleTime=-1  HasFrameUpgradeWarning=on
  i_beta_hat : Outport
  wires:
  Gain8/1 -> Add1/2
  u_beta/1 -> Gain5/1
  Add1/1 -> Integrator1/1
  Gain3/1 -> Add1/3
  i_alpha_hat/1 -> Product1/1
  Gain5/1 -> Add1/4
  Gain6/1 -> Add1/5
  Integrator1/1 -> Unit Delay1/1
  Product1/1 -> Gain7/1
  Gain7/1 -> Add1/1
  beta_err/1 -> Gain6/1
  e_beta_hat/1 -> Gain3/1
  Unit Delay1/1 -> [I_beta_hat], i_beta_hat/1
  omega_hat/1 -> Product1/2
  [I_beta_hat] -> Gain8/1

== system PMSM_FOC_Traction/Motor_Control/Motor_Control_Funtion/Angle_Speed_100us/HIGH_SMO/Equ3 ==
  note: GainM/Ld
  note: e_alpha_hat_dot
  omega_hat : Inport
  e_beta_hat : Inport  Port=2
  alpha_err : Inport  Port=3
  Add2 : Sum  Inputs=-+
  Gain9 : Gain  Gain=SMO.m/pmsm.InductanceLd
  Integrator2 : DiscreteIntegrator  IntegratorMethod=Integration: Backward Euler  SampleTime=-1  ICPrevOutput=DiscIntNeverNeededParam  ICPrevScaledInput=DiscIntNeverNeededParam  mask(DiscretizedDiscreteIntegrator){}
      mask init:
      | %tustin
  Product2 : Product
  Unit Delay2 : UnitDelay  SampleTime=-1  HasFrameUpgradeWarning=on
  e_alpha_hat : Outport
  wires:
  alpha_err/1 -> Gain9/1
  Add2/1 -> Integrator2/1
  Unit Delay2/1 -> e_alpha_hat/1
  omega_hat/1 -> Product2/1
  Product2/1 -> Add2/1
  Integrator2/1 -> Unit Delay2/1
  e_beta_hat/1 -> Product2/2
  Gain9/1 -> Add2/2

== system PMSM_FOC_Traction/Motor_Control/Motor_Control_Funtion/Angle_Speed_100us/HIGH_SMO/Equ4 ==
  note: GainM/Ld
  note: e_beta_hat_dot
  omega_hat : Inport
  e_alpha_hat : Inport  Port=2
  beta_err : Inport  Port=3
  Add3 : Sum
  Gain10 : Gain  Gain=SMO.m/pmsm.InductanceLd
  Integrator3 : DiscreteIntegrator  IntegratorMethod=Integration: Backward Euler  SampleTime=-1  ICPrevOutput=DiscIntNeverNeededParam  ICPrevScaledInput=DiscIntNeverNeededParam  mask(DiscretizedDiscreteIntegrator){}
      mask init:
      | %tustin
  Product3 : Product
  Unit Delay3 : UnitDelay  SampleTime=-1  HasFrameUpgradeWarning=on
  e_beta_hat : Outport
  wires:
  Integrator3/1 -> Unit Delay3/1
  Add3/1 -> Integrator3/1
  Gain10/1 -> Add3/2
  Product3/1 -> Add3/1
  beta_err/1 -> Gain10/1
  Unit Delay3/1 -> e_beta_hat/1
  omega_hat/1 -> Product3/1
  e_alpha_hat/1 -> Product3/2

== system PMSM_FOC_Traction/Motor_Control/Motor_Control_Funtion/Angle_Speed_100us/HIGH_SMO/QPLL ==
  e_alpha_hat : Inport
  e_beta_hat : Inport  Port=2
  Cos1 : Trigonometry  Operator=cos
  PIDTheta_Ctrl : pid_lib/PID Controller  Controller=PI  Form=Parallel  TimeDomain=Discrete-time  UseExternalTs=off  SampleTime=-1  IntegratorMethod=Forward Euler  FilterMethod=Forward Euler  ControllerParametersSource=internal  P=2*0.707*100  I=100*100  D=0  UseFilter=on  N=100  TunerSelectOption=Transfer Function Based (PID Tuner App)  ZeroCross=off  InitialConditionSource=internal  InitialConditionForIntegrator=1  InitialConditionForFilter=0  DifferentiatorICPrevScaledInput=0  ExternalReset=none  TrackingMode=off  Kt=1  LimitOutput=on  SatLimitsSource=internal  UpperSaturationLimit=2*pi*500  LowerSaturationLimit=-2*pi*500  LinearizeAsGain=off  AntiWindupMode=clamping  Kb=50  POutMin=[]  POutMax=[]  IOutMin=[]  IOutMax=[]  DOutMin=[]  DOutMax=[]  NOutMin=[]  NOutMax=[]  SumOutMin=[]  SumOutMax=[]  SaturationOutDataTypeStr=Inherit: Inherit via back propagation  SaturationOutMin=[]  SaturationOutMax=[]  PParamMin=[]  PParamMax=[]  IParamMin=[]  IParamMax=[]  DParamMin=[]  DParamMax=[]  NParamMin=[]  NParamMax=[]  KbParamMin=[]  KbParamMax=[]  KtParamMin=[]  KtParamMax=[]  KbOutMin=[]  KbOutMax=[]  KtOutMin=[]  KtOutMax=[]  IntegratorOutMin=[]  IntegratorOutMax=[]  FilterOutMin=[]  FilterOutMax=[]  SumI1OutMin=[]  SumI1OutMax=[]  SumI2OutMin=[]  SumI2OutMax=[]  SumI3OutMin=[]  SumI3OutMax=[]  SumI4OutMin=[]  SumI4OutMax=[]  SumDOutMin=[]  SumDOutMax=[]  DifferentiatorOutMin=[]  DifferentiatorOutMax=[]  FilterDiffOutCoefMin=[]  FilterDiffOutCoefMax=[]  ReciprocalOutMin=[]  ReciprocalOutMax=[]  SumDenOutMin=[]  SumDenOutMax=[]  SumNumOutMin=[]  SumNumOutMax=[]  DivideOutMin=[]  DivideOutMax=[]  UdiffTsProdOutMin=[]  UdiffTsProdOutMax=[]  NTsProdOutMin=[]  NTsProdOutMax=[]  UintegralTsProdOutMin=[]  UintegralTsProdOutMax=[]  UngainTsProdOutMin=[]  UngainTsProdOutMax=[]  IntegratorContinuousStateAttributes=''  IntegratorStateMustResolveToSignalObject=off  IntegratorRTWStateStorageClass=Auto  FilterContinuousStateAttributes=''  FilterStateMustResolveToSignalObject=off  FilterRTWStateStorageClass=Auto  ParallelPVariant=InternalParameters  IdealPVariant=Disabled  IVariant=InternalParameters  DVariant=Disabled  IntegratorVariant=Discrete  SatVariant=Enabled  AWVariant=DiscClampingParallel  PCopyVariant=Disabled  TRVariant=Disabled  FdbkBlocksVariant=Forward  IdealPFdbkVariant=Disabled  SatFdbkVariant=Disabled  DerivativeFilterVariant=Disabled  NVariant=Disabled  NCopyVariant=Disabled_SignalSpec  FilterICVariant=Disabled  IntegratorICVariant=InternalICs  ExternalResetVariant=Disabled  TRSumVariant=Passthrough  SumFdbkVariant=Disabled  SumVariant=Sum_PI  TsampFilterVariant=InternalTs  TsampNgainVariant=Passthrough  TsampIntegralVariant=Passthrough  ExternalSaturationOutDataTypeStr=Inherit: Same as second input
  Product1 : Product
  Product2 : Product
  Sin1 : Trigonometry
  SpeedToTheta : Subsystem
  Subsystem1 : Subsystem
  Sum : Sum  Inputs=|--
  Unit Delay : UnitDelay  SampleTime=-1  HasFrameUpgradeWarning=on
  sin_cos : Outport
  speed_hat : Outport  Port=2
  wires:
  Sin1/1 -> Product1/2
  Subsystem1/1(Out) -> PIDTheta_Ctrl/1
  Cos1/1 -> Product2/1
  Sum/1 -> Subsystem1/1(Err_in)
  Product1/1 -> Sum/2
  Product2/1 -> Sum/1
  e_beta_hat/1 -> Product1/1
  e_alpha_hat/1 -> Product2/2
  Unit Delay/1 -> speed_hat/1, Subsystem1/2(speed)  "speed_hat"
  [theta_hat] -> Sin1/1
  [theta_hat] -> Cos1/1
  PIDTheta_Ctrl/1 -> Unit Delay/1, SpeedToTheta/1(In1)
  SpeedToTheta/1(sin_cos) -> sin_cos/1, [theta_hat]

== system PMSM_FOC_Traction/Motor_Control/Motor_Control_Funtion/Angle_Speed_100us/Resolver_Observer/Angle_calibration ==
  Angle_input : Inport
  Angle_offset : Constant  Value=Resolver_Parameter.PLL_Angle_offset
  If Action Subsystem1 : Subsystem  TreatAsAtomicUnit=on
  If Action Subsystem2 : Subsystem  TreatAsAtomicUnit=on
  If Action Subsystem3 : Subsystem  TreatAsAtomicUnit=on
  If1 : If  IfExpression=u1 > 6.283185307  ElseIfExpressions=u1<0
  Merge1 : Merge  Inputs=3
  Subtract1 : Sum
  Angle_output : Outport
  wires:
  If1/2 -> If Action Subsystem3/Action
  If Action Subsystem1/1(Out1) -> Merge1/3
  If1/3 -> If Action Subsystem1/Action
  If Action Subsystem3/1(Out1) -> Merge1/2
  If Action Subsystem2/1(Out1) -> Merge1/1
  Subtract1/1 -> If Action Subsystem3/1(In1), If Action Subsystem1/1(In1), If Action Subsystem2/1(In1), If1/1
  If1/1 -> If Action Subsystem2/Action
  Angle_offset/1 -> Subtract1/2
  Angle_input/1 -> Subtract1/1
  Merge1/1 -> Angle_output/1

== system PMSM_FOC_Traction/Motor_Control/Motor_Control_Funtion/Angle_Speed_100us/Resolver_Observer/Resolver_Angle_cacl ==
  Sin_Cos : Inport
  2*pi : Constant  Value=2*pi  OutDataTypeStr=single  SampleTime=-1
  B : Selector  IndexMode=Zero-based  InputPortWidth=2  IndexOptions=Index vector (dialog)  Indices=0  OutputSizes=1
  C : Selector  IndexMode=Zero-based  InputPortWidth=2  IndexOptions=Index vector (dialog)  Indices=1  OutputSizes=1
  Constant : Constant  OutDataTypeStr=single  SampleTime=-1
  Discrete-Time Integrator : DiscreteIntegrator  SampleTime=-1  ICPrevOutput=DiscIntNeverNeededParam  ICPrevScaledInput=DiscIntNeverNeededParam
  Gain : Gain  Gain=15/(2*pi)
  LPF : DiscreteFilter  Numerator=[0 0.04]  Denominator=[1 -0.96]
  Math Function : Math  Operator=mod  SignedPower=on  SaturateOnIntegerOverflow=on
  PID Controller : pid_lib/PID Controller  Controller=PI  Form=Parallel  TimeDomain=Discrete-time  UseExternalTs=off  SampleTime=-1  IntegratorMethod=Forward Euler  FilterMethod=Forward Euler  ControllerParametersSource=internal  P=141  I=10000  D=0  UseFilter=off  N=100  TunerSelectOption=Transfer Function Based (PID Tuner App)  InitialConditionSource=internal  InitialConditionForIntegrator=0  InitialConditionForFilter=0  DifferentiatorICPrevScaledInput=0  ExternalReset=none  TrackingMode=off  Kt=1  LimitOutput=off  SatLimitsSource=internal  UpperSaturationLimit=inf  LowerSaturationLimit=-inf  LinearizeAsGain=on  AntiWindupMode=none  Kb=1  POutMin=[]  POutMax=[]  IOutMin=[]  IOutMax=[]  DOutMin=[]  DOutMax=[]  NOutMin=[]  NOutMax=[]  SumOutMin=[]  SumOutMax=[]  SaturationOutMin=[]  SaturationOutMax=[]  PParamMin=[]  PParamMax=[]  IParamMin=[]  IParamMax=[]  DParamMin=[]  DParamMax=[]  NParamMin=[]  NParamMax=[]  KbParamMin=[]  KbParamMax=[]  KtParamMin=[]  KtParamMax=[]  KbOutMin=[]  KbOutMax=[]  KtOutMin=[]  KtOutMax=[]  IntegratorOutMin=[]  IntegratorOutMax=[]  FilterOutMin=[]  FilterOutMax=[]  SumI1OutMin=[]  SumI1OutMax=[]  SumI2OutMin=[]  SumI2OutMax=[]  SumI3OutMin=[]  SumI3OutMax=[]  SumI4OutMin=[]  SumI4OutMax=[]  SumDOutMin=[]  SumDOutMax=[]  DifferentiatorOutMin=[]  DifferentiatorOutMax=[]  FilterDiffOutCoefMin=[]  FilterDiffOutCoefMax=[]  ReciprocalOutMin=[]  ReciprocalOutMax=[]  SumDenOutMin=[]  SumDenOutMax=[]  SumNumOutMin=[]  SumNumOutMax=[]  DivideOutMin=[]  DivideOutMax=[]  UdiffTsProdOutMin=[]  UdiffTsProdOutMax=[]  NTsProdOutMin=[]  NTsProdOutMax=[]  UintegralTsProdOutMin=[]  UintegralTsProdOutMax=[]  UngainTsProdOutMin=[]  UngainTsProdOutMax=[]  IntegratorContinuousStateAttributes=''  IntegratorStateMustResolveToSignalObject=off  IntegratorRTWStateStorageClass=Auto  FilterContinuousStateAttributes=''  FilterStateMustResolveToSignalObject=off  FilterRTWStateStorageClass=Auto  ParallelPVariant=InternalParameters  IdealPVariant=Disabled  IVariant=InternalParameters  DVariant=Disabled  IntegratorVariant=Discrete  SatVariant=Disabled  AWVariant=Passthrough  PCopyVariant=Disabled  TRVariant=Disabled  FdbkBlocksVariant=Forward  IdealPFdbkVariant=Disabled  SatFdbkVariant=Disabled  DerivativeFilterVariant=Disabled  NVariant=Disabled  NCopyVariant=Disabled_SignalSpec  FilterICVariant=Disabled  IntegratorICVariant=InternalICs  ExternalResetVariant=Disabled  TRSumVariant=Passthrough  SumFdbkVariant=Disabled  SumVariant=Sum_PI  TsampFilterVariant=InternalTs  TsampNgainVariant=Passthrough  TsampIntegralVariant=Passthrough  ExternalSaturationOutDataTypeStr=Inherit: Same as second input
  Product : Product  OutDataTypeStr=single
  Product{1..4} (4 alike) : Product
  Scope : Scope  NumInputPorts=2
  Scope{1,3..4,6..7} (5 alike) : Scope
  Scope2 : Scope  NumInputPorts=2
  Scope5 : Scope  NumInputPorts=2
  Sine_Cosine : Subsystem  TreatAsAtomicUnit=on
      settings: RTWSystemCode=Nonreusable function  RTWFcnNameOpts=Use subsystem name
  Sum1 : Sum  Inputs=-+
  Unit Delay4 : UnitDelay  SampleTime=-1  HasFrameUpgradeWarning=on
  constant : Constant  OutDataTypeStr=single
  "pole pairs " : Gain  OutDataTypeStr=single
  Velocity : Outport  VectorParamsAs1DForOutWhenUnconnected=off
  Angle : Outport  Port=2  VectorParamsAs1DForOutWhenUnconnected=off
  wires:
  Product2/1 -> Scope2/2, Product4/1
  Product4/1 -> Scope/2, Sum1/2
  Sin_Cos/1 -> C/1, B/1
  Unit Delay4/1 -> Product/2
  Sum1/1 -> PID Controller/1
  Product3/1 -> Scope/1, Sum1/1
  Constant/1 -> Product/1
  constant/1 -> Product2/1, Product1/1
  Product/1 -> Sine_Cosine/1(P)
  Sine_Cosine/1(Sin) -> Product1/2
  Product1/1 -> Scope2/1, Product3/2
  Math Function/1 -> Unit Delay4/1, Angle/1, Scope4/1  "Angle_Theta"
  Gain/1 -> LPF/1, Scope3/1  "Speed_RPM"
  Discrete-Time Integrator/1 -> Scope6/1, "pole pairs "/1
  "pole pairs "/1 -> Math Function/1
  PID Controller/1 -> Discrete-Time Integrator/1, Gain/1
  2*pi/1 -> Math Function/2
  B/1 -> Scope1/1, Product3/1, Scope5/2, Scope5/1  "Vx"
  C/1 -> Product4/2, Scope7/1  "Vy"
  LPF/1 -> Velocity/1
  Sine_Cosine/2(Cos) -> Product2/2

== system PMSM_FOC_Traction/Motor_Control/Motor_Control_Funtion/Angle_Speed_100us/SMO/Angle_calibration ==
  Angle_input : Inport
  Angle_offset : Constant  Value=SMO.Angle_offset
  If Action Subsystem1 : Subsystem  TreatAsAtomicUnit=on
  If Action Subsystem2 : Subsystem  TreatAsAtomicUnit=on
  If Action Subsystem3 : Subsystem  TreatAsAtomicUnit=on
  If1 : If  IfExpression=u1 > 6.283185307  ElseIfExpressions=u1<0
  Merge1 : Merge  Inputs=3
  Subtract1 : Sum
  Angle_output : Outport
  wires:
  Angle_input/1 -> Subtract1/1
  Angle_offset/1 -> Subtract1/2  "Control_ModeCommand"
  If1/1 -> If Action Subsystem2/Action
  If1/3 -> If Action Subsystem1/Action
  If Action Subsystem2/1(Out1) -> Merge1/1
  Subtract1/1 -> If Action Subsystem3/1(In1), If Action Subsystem1/1(In1), If Action Subsystem2/1(In1), If1/1
  If Action Subsystem1/1(Out1) -> Merge1/3
  If Action Subsystem3/1(Out1) -> Merge1/2
  If1/2 -> If Action Subsystem3/Action
  Merge1/1 -> Angle_output/1
